simulink model "LoadFlow58BusNetwork_2023"  (R2023b)
settings: Solver=FixedStepDiscrete  StartTime=0.0  StopTime=4.5  FixedStep=75e-6  RelTol=1e-3  EnableMultiTasking=on
undefined symbols (not defined in the file): D1, D11, Delta
libraries: spsSeriesRLCBranchLib x41, spsLoadFlowBusLib x29, spsDistributedParametersLineLib x19, spsThreePhaseSeriesRLCLoadLib x15, spsThreePhaseTransformerTwoWindingsLib x13, spsThreePhaseParallelRLCLoadLib x11, spsThreePhaseVIMeasurementLib x11, spsSynchronousMachinepuStandardLib x7, spsExcitationSystemLib x7, spsHydraulicTurbineandGovernorLib x7, spsGenericPowerSystemStabilizerLib x7, spsMultiBandPowerSystemStabilizerLib x7
(part 3 of 5)

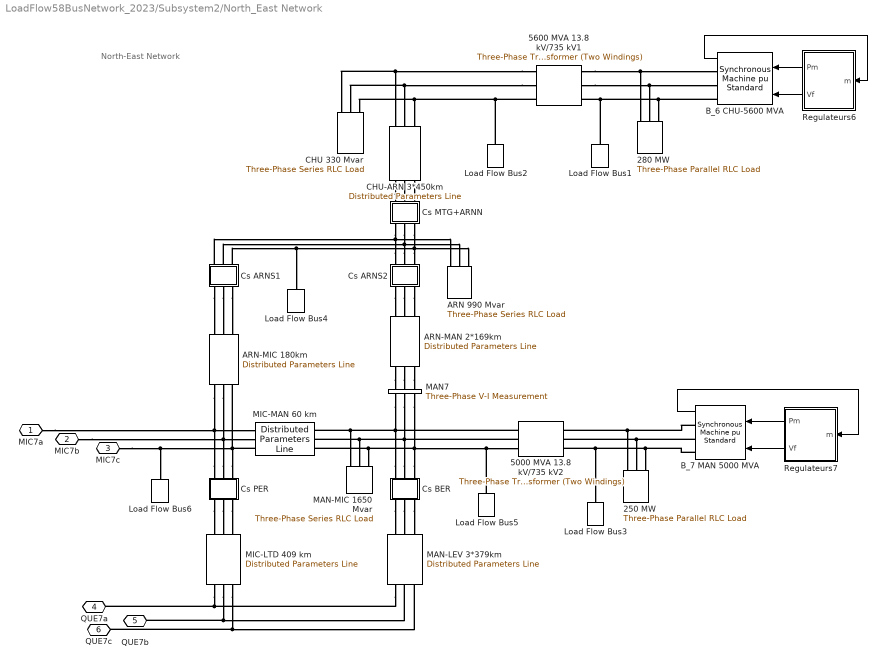
== system LoadFlow58BusNetwork_2023/Subsystem2/North_East Network ==
  note: North-East Network
  250 MW : spsThreePhaseParallelRLCLoadLib/Three-Phase Parallel RLC Load  LConnTagsString=A|B|C  Configuration=Y (grounded)  NominalVoltage=(13800)*1  Vabc=[1e3 1e3 1e3]  Vabcp=[1e3 1e3 1e3]  NominalFrequency=60  UnbalancedPower=off  ActivePower=250000000  InductivePower=0  CapacitivePower=0  Pabc=[10e3 9e3 11e3]  QLabc=[100 90 110]  QCabc=[100 90 110]  Pabcp=[10e3 9e3 11e3]  QLabcp=[100 90 110]  QCabcp=[100 90 110]  Measurements=None  LoadType=constant PQ
  280 MW : spsThreePhaseParallelRLCLoadLib/Three-Phase Parallel RLC Load  LConnTagsString=A|B|C  Configuration=Y (grounded)  NominalVoltage=(13800)*1  Vabc=[1e3 1e3 1e3]  Vabcp=[1e3 1e3 1e3]  NominalFrequency=60  UnbalancedPower=off  ActivePower=280000000  InductivePower=0  CapacitivePower=0  Pabc=[10e3 9e3 11e3]  QLabc=[100 90 110]  QCabc=[100 90 110]  Pabcp=[10e3 9e3 11e3]  QLabcp=[100 90 110]  QCabcp=[100 90 110]  Measurements=None  LoadType=constant PQ
  5000 MVA 13.8 kV/735 kV2 : spsThreePhaseTransformerTwoWindingsLib/Three-Phase Transformer (Two Windings)  Winding1Connection=Delta (D1)  Winding2Connection=Yg  CoreType=Three single-phase transformers  SetSaturation=off  Hysteresis=off  DataFile='basic_model'  SetInitialFlux=off  Measurements=None  UNITS=pu  NominalPower=[ 5000e6 60 ]  Winding1="[ 13.8e3 0.002  0.0]"  Winding2=[ 735e3 0.002 0.12]  Rm=500  Lm=500  L0=0.5  Saturation="[ 0,0  ;  0.005,1.2  ;  1.0,1.4 ]"  InitialFluxes=[ 0.8 , -0.8 , 0.7 ]  BreakLoop=off  DiscreteSolver=Trapezoidal iterative  DataType=off  TransfoNumber=0
  5600 MVA 13.8 kV/735 kV1 : spsThreePhaseTransformerTwoWindingsLib/Three-Phase Transformer (Two Windings)  Winding1Connection=Delta (D1)  Winding2Connection=Yg  CoreType=Three single-phase transformers  SetSaturation=off  Hysteresis=off  DataFile='basic_model'  SetInitialFlux=off  Measurements=None  UNITS=pu  NominalPower=[ 5600e6 60 ]  Winding1="[ 13.8e3 0.002  0.0]"  Winding2=[ 735e3 0.002 0.12]  Rm=500  Lm=500  L0=0.5  Saturation="[ 0,0  ;  0.005,1.2  ;  1.0,1.4 ]"  InitialFluxes=[ 0.8 , -0.8 , 0.7 ]  BreakLoop=off  DiscreteSolver=Trapezoidal iterative  DataType=off  TransfoNumber=0
  ARN 990 Mvar : spsThreePhaseSeriesRLCLoadLib/Three-Phase Series RLC Load  LConnTagsString=A|B|C  Configuration=Y (grounded)  NominalVoltage=735e3  Vabc=[1e3 1e3 1e3]  Vabcp=[1e3 1e3 1e3]  NominalFrequency=60  UnbalancedPower=off  ActivePower=3300000  InductivePower=990e6  CapacitivePower=0  Pabc=[10e3 9e3 11e3]  QLabc=[100 90 110]  QCabc=[100 90 110]  Pabcp=[10e3 9e3 11e3]  QLabcp=[100 90 110]  QCabcp=[100 90 110]  Measurements=None  LoadType=constant Z
  ARN-MAN 2*169km : spsDistributedParametersLineLib/Distributed Parameters Line  Phases=3  Length=169  Frequency=60  Resistance="[0.01273  0.3864]/2"  Inductance="[0.9337e-3  4.1264e-3]/2"  Capacitance=[12.74e-9 7.751e-9]*2  x1=[-0.000975 1.67050882449748e-09 347873.977312553 -681165.145140791;-0.0009 1.59985900326383e-09 366991.883229444 -671058.367402093;-0.000825 1.52793027922164e-09 385816.421450045 -660415.155872031;-0.00075 1.45478015109235e-09 404332.543926528 -649244.018571055;-0.000675 1.38046709396916e-09 422525.449153892 -637553.8855354;-0.0006 1.30505051257291e-09 440380.594002059 -625354.10167855;-0.000525 1.22859069376485e-09 457883.705341429 -612654.419321056;-0.00045 1.15114875835426e-09 475020.791452605 -599464.990394684;-0.000375 1.07278661223941e-09 491778.153211155 -585796.358327113;-0.0003 9.93566896920918e-10 508142.395038487 -571659.44961368;-0.000225 9.13552939427113e-10 524100.435610064 -557065.565082908;-0.00015 8.3280870169136e-10 539639.51831242 -542026.370862799;-7.5e-05 7.51398729421874e-10 554747.221440599 -526553.889055102]  x2=[-0.000975 1.50504449601884e-09 232985.418240298 -689450.364518884;-0.0009 1.46263645773588e-09 252383.458947633 -682588.200672076;-0.000825 1.41905921024769e-09 271579.748179482 -675180.3862616;-0.00075 1.37434758853916e-09 290558.940715946 -667232.842980953;-0.000675 1.32853733439658e-09 309305.864880903 -658751.923974632;-0.0006 1.28166506783619e-09 327805.534670012 -649744.408759529;-0.000525 1.2337682578307e-09 346043.161730299 -640217.497805485;-0.00045 1.18488519235719e-09 364004.167181736 -630178.806779352;-0.000375 1.13505494779026e-09 381674.193271379 -619636.360457139;-0.0003 1.08431735766499e-09 399039.114850732 -608598.586309131;-0.000225 1.03271298083461e-09 416085.050667176 -597074.307763098;-0.00015 9.80283069048393e-10 432798.374460432 -585072.737150982;-7.5e-05 9.27069533975612e-10 449165.725855181 -572603.4683447]  x3=[-0.000975 -5.34124314733807e-12 1583.75858462539 -1421.24992657659;-0.0009 -5.43018616572326e-12 1623.30400424483 -1375.9090252372;-0.000825 -5.5147883763722e-12 1661.55177948066 -1329.46824327516;-0.00075 -5.59498214957216e-12 1698.47133564656 -1281.96470474099;-0.000675 -5.67070337964786e-12 1734.03315981423 -1233.43638323657;-0.0006 -5.74189153620653e-12 1768.20882440555 -1183.9220715596;-0.000525 -5.80848971252505e-12 1800.97100991713 -1133.46135069323;-0.00045 -5.87044467104025e-12 1832.29352675917 -1082.09455816567;-0.000375 -5.92770688590623e-12 1862.15133619095 -1029.86275580491;-0.0003 -5.98023058258458e-12 1890.52057033645 -976.807696914584;-0.000225 -6.0279737744358e-12 1917.37855126396 -922.971792897006;-0.00015 -6.07089829628284e-12 1942.70380911446 -868.398079350128;-7.5e-05 -6.10896983491968e-12 1966.47609926432 -813.130181665554]  x4=[-0.000975 9.21214000394156e-12 1569.30174481224 -9115.59279820432;-0.0009 9.04527834437803e-12 1826.37892659041 -9067.5841614058;-0.000825 8.87118602770341e-12 2081.9961289992 -9012.32703656734;-0.00075 8.69000222065193e-12 2335.94901555807 -8949.86559538908;-0.000675 8.50187175878676e-12 2588.03458021512 -8880.2497685914;-0.0006 8.30694503072062e-12 2838.05130962701 -8803.53520600108;-0.000525 8.10537785789743e-12 3085.79934424562 -8719.78323206569;-0.00045 7.89733137003109e-12 3331.08063808276 -8629.06079683175;-0.000375 7.68297187630076e-12 3573.69911702505 -8531.44042242588;-0.0003 7.46247073240593e-12 3813.46083557263 -8427.00014508173;-0.000225 7.23600420358725e-12 4050.17413187616 -8315.82345275904;-0.00015 7.0037533237228e-12 4283.6497809484 -8197.99921840457;-7.5e-05 6.76590375061238e-12 4513.7011459278 -8073.62162890851]  x5=0.000955765248222805  V1=ones(3,3)  V2=ones(3,3)  I1=ones(3,3)  I2=ones(3,3)  nHarmo=1  Measurements=None  Decoupling=on  VsMag0=[624500.54274601 624501.904306242 624500.0432619]  VrMag0=[594207.380493356 594208.101305703 594207.286862308]  VsAngle0=[18.1135948354225 -101.886530201485 138.113424134242]  VrAngle0=[9.73160889879617 -110.268441654027 129.731523430545]  IsMag0=[1744.35611857334 1744.39210598387 1744.37536737728]  IrMag0=[7582.44376493461 7582.4337899273 7582.40838117022]  IsAngle0=[39.1559168024789 -80.8440356055226 159.154916919434]  IrAngle0=[0.828149284036499 -119.172115933984 120.828081951982]
      settings: AttributesFormatString=\n  LibrarySourceBlock=sps_lib/Power Grid Elements/Distributed Parameters Line
  ARN-MIC 180km : spsDistributedParametersLineLib/Distributed Parameters Line  Phases=3  Length=180  Frequency=60  Resistance="[0.01273  0.3864]"  Inductance="[0.9337e-3  4.1264e-3]"  Capacitance=[12.74e-9 7.751e-9]  x1=[-0.00105 1.27410114359668e-09 336203.730988153 -674396.62729794;-0.000975 1.20660459291676e-09 355134.952563368 -664622.476598216;-0.0009 1.13814350098693e-09 373782.284691251 -654317.036859764;-0.000825 1.0687725945566e-09 392130.820979812 -643488.546093432;-0.00075 9.98547327666939e-10 410165.893889885 -632145.660429059;-0.000675 9.27523837321831e-10 427873.086460132 -620297.447195891;-0.0006 8.5575889861276e-10 445238.243831739 -607953.377674304;-0.000525 7.83309879333687e-10 462247.484563601 -595123.319524603;-0.00045 7.10234694122118e-10 478887.211728927 -581817.528898967;-0.000375 6.36591758163024e-10 495144.123784416 -568046.642242835;-0.0003 5.62439940492634e-10 511005.225203312 -553821.667792299;-0.000225 4.87838516939434e-10 526457.836863822 -539153.976774286;-0.00015 4.12847122739972e-10 541489.606184618 -524055.294316571;-7.5e-05 3.37525704867365e-10 556088.516999299 -508537.690074895]  x2=[-0.00105 4.36302610467453e-09 192165.57848685 -719334.039084997;-0.000975 4.3093865404647e-09 212424.764832704 -713613.931123378;-0.0009 4.25230211859025e-09 232514.142071759 -707323.371103878;-0.000825 4.1918184714646e-09 252417.651063227 -700467.387603928;-0.00075 4.12798394878983e-09 272119.381246555 -693051.461191837;-0.000675 4.06084957890668e-09 291603.583360081 -685081.520045713;-0.0006 3.99046902800322e-09 310854.682030753 -676563.935214563;-0.000525 3.91689855721501e-09 329857.288224845 -667505.515525378;-0.00045 3.84019697765071e-09 348596.211549717 -657913.502140259;-0.000375 3.76042560337947e-09 367056.472396776 -647795.562767943;-0.0003 3.67764820241733e-09 385223.313915954 -637159.785534355;-0.000225 3.59193094575207e-09 403082.213812102 -626014.672517082;-0.00015 3.50334235444717e-09 420618.895953893 -614369.132948945;-7.5e-05 3.41195324486706e-09 437819.341785944 -602232.476096092]  x3=[-0.00105 3.66209367040117e-12 149.00166074947 -364.54093553914;-0.000975 3.89569353874418e-12 159.247423691884 -360.183291873256;-0.0009 4.12617924927843e-12 169.365886680365 -355.537723194838;-0.000825 4.35336655525346e-12 179.348961170419 -350.607943100407;-0.00075 4.57707384661297e-12 189.188666845044 -345.397892380743;-0.000675 4.79712229517107e-12 198.877137994077 -339.911735870675;-0.0006 5.01333599756484e-12 208.406629801921 -334.153859119776;-0.000525 5.22554211586878e-12 217.769524538628 -328.128864886622;-0.00045 5.43357101575876e-12 226.958337649405 -321.841569459417;-0.000375 5.63725640211517e-12 235.965723737644 -315.296998805928;-0.0003 5.83643545195665e-12 244.784482436724 -308.5003845558;-0.000225 6.03094894459828e-12 253.407564165872 -301.457159818471;-0.00015 6.22064138893022e-12 261.828075765492 -294.172954840033;-7.5e-05 6.40536114771486e-12 270.039286007448 -286.653592502493]  x4=[-0.00105 4.34965354391857e-12 1187.65933351948 -4979.46515427095;-0.000975 3.97419055552239e-12 1327.95758028668 -4943.89904376724;-0.0009 3.59555066000328e-12 1467.19427808263 -4904.38085601213;-0.000825 3.21403653630033e-12 1605.25812322151 -4860.94218124028;-0.00075 2.82995316096667e-12 1742.03874957796 -4813.61774366365;-0.000675 2.44360756437587e-12 1877.42681681208 -4762.44537371355;-0.0006 2.05530858528656e-12 2011.31409777444 -4707.46597779957;-0.000525 1.66536662396144e-12 2143.59356502117 -4648.72350560958;-0.00045 1.27409339403809e-12 2274.15947637011 -4586.26491497706;-0.000375 8.81801673349837e-13 2402.90745942944 -4520.14013434371;-0.0003 4.88805053895921e-13 2529.73459503142 -4450.40202284743;-0.000225 9.54176911608898e-14 2654.53949950437 -4377.10632806753;-0.00015 -2.98045947016516e-13 2777.22240571723 -4300.31164146093;-7.5e-05 -6.91271331824133e-13 2897.6852428319 -4220.07935152513]  x5=0.00101797482059234  V1=ones(3,3)  V2=ones(3,3)  I1=ones(3,3)  I2=ones(3,3)  nHarmo=1  Measurements=None  Decoupling=on  VsMag0=[615273.936100182 615275.237959051 615273.425867036]  VrMag0=[607930.231675994 607930.97680853 607930.152146888]  VsAngle0=[19.1774103741915 -100.822714483789 139.177242954875]  VrAngle0=[7.63692875074741 -112.363120449619 127.636843332413]  IsMag0=[322.896150601901 322.910343515413 322.909058922171]  IrMag0=[4197.50413399043 4197.49907033619 4197.48826872784]  IsAngle0=[14.9112658694072 -105.087543385455 134.90968031067]  IrAngle0=[6.09512812442914 -113.905082032173 126.095082904965]
      settings: AttributesFormatString=\n  LibrarySourceBlock=sps_lib/Power Grid Elements/Distributed Parameters Line
  "B_6 CHU-5600 MVA " : spsSynchronousMachinepuStandardLib/Synchronous Machine pu Standard  PresetModel=No  MechanicalLoad=Mechanical power Pm  ShowDetailedParameters=on  RotorType=Salient-pole  Units=per unit standard parameters  MeasurementBus=off  NominalParameters="[ 5600E6  13800   60 ]"  Reactances1=[ 31 32 33 34 35 36 37 ]  Reactances2=[ 1.305, 0.296, 0.252, 0.474, 0.243, 0.18 ]  dAxisTimeConstants=Short-circuit  qAxisTimeConstants=Open-circuit  TimeConstants1=[]  TimeConstants2=[]  TimeConstants3=[]  TimeConstants4=[]  TimeConstants5=[ 1.01, 0.053, 0.1 ]  TimeConstants6=[]  TimeConstants7=[]  TimeConstants8=[]  StatorResistance=2.8544e-3  Mechanical="[ 4.0 0  32]"  PolePairs=32  InitialConditions=[0 -61.7964 0.894782 0.894782 0.894782 8.48442 -111.516 128.484 1.31361]  SetSaturation=off  Saturation=[0.6404,0.7127,0.8441,0.9214,0.9956,1.082,1.19,1.316,1.457;0.7,0.7698,0.8872,0.9466,0.9969,1.046,1.1,1.151,1.201]  LoadFlowParameters=[1 5000000000 0 0 0]  TsPowergui=0  TsBlock=-1  IterativeModel=Trapezoidal non iterative  IterativeDiscreteModel=Trapezoidal non iterative  BusType=PV  Pref=5000000000  Qref=0  Qmin=-Inf  Qmax=Inf  PLF=0  QLF=0
  B_7 MAN 5000 MVA : spsSynchronousMachinepuStandardLib/Synchronous Machine pu Standard  PresetModel=No  MechanicalLoad=Mechanical power Pm  ShowDetailedParameters=on  RotorType=Salient-pole  Units=per unit standard parameters  MeasurementBus=off  NominalParameters="[ 5000E6  13800   60 ]"  Reactances1=[ 31 32 33 34 35 36 37 ]  Reactances2=[ 1.305, 0.296, 0.252, 0.474, 0.243, 0.18 ]  dAxisTimeConstants=Short-circuit  qAxisTimeConstants=Open-circuit  TimeConstants1=[]  TimeConstants2=[]  TimeConstants3=[]  TimeConstants4=[]  TimeConstants5=[ 1.01, 0.053, 0.1 ]  TimeConstants6=[]  TimeConstants7=[]  TimeConstants8=[]  StatorResistance=2.8544e-3  Mechanical="[ 3.7 0  32]"  PolePairs=32  InitialConditions=[0 -81.9543 0.907703 0.907703 0.907703 -8.76021 -128.76 111.24 1.25655]  SetSaturation=off  Saturation=[0.6404,0.7127,0.8441,0.9214,0.9956,1.082,1.19,1.316,1.457;0.7,0.7698,0.8872,0.9466,0.9969,1.046,1.1,1.151,1.201]  LoadFlowParameters=[1 4500000000 0 0 0]  TsPowergui=0  TsBlock=-1  IterativeModel=Trapezoidal non iterative  IterativeDiscreteModel=Trapezoidal non iterative  BusType=PV  Pref=4500000000  Qref=0  Qmin=-Inf  Qmax=Inf  PLF=0  QLF=0
  CHU 330 Mvar : spsThreePhaseSeriesRLCLoadLib/Three-Phase Series RLC Load  LConnTagsString=A|B|C  Configuration=Y (grounded)  NominalVoltage=735e3  Vabc=[1e3 1e3 1e3]  Vabcp=[1e3 1e3 1e3]  NominalFrequency=60  UnbalancedPower=off  ActivePower=1100000  InductivePower=330e6  CapacitivePower=0  Pabc=[10e3 9e3 11e3]  QLabc=[100 90 110]  QCabc=[100 90 110]  Pabcp=[10e3 9e3 11e3]  QLabcp=[100 90 110]  QCabcp=[100 90 110]  Measurements=None  LoadType=constant Z
  CHU-ARN 3*450km : spsDistributedParametersLineLib/Distributed Parameters Line  Phases=3  Length=450  Frequency=60  Resistance="[0.01273  0.3864]/3"  Inductance="[0.9337e-3  4.1264e-3]/3"  Capacitance=[12.74e-9 7.751e-9]*3  x1=[-0.00255 1.72762635052858e-09 0 0;-0.002475 1.64166254069958e-09 0 0;-0.0024 1.55438641095382e-09 0 0;-0.002325 1.46586772849405e-09 0 0;-0.00225 1.37617725380066e-09 0 0;-0.002175 1.28538668406679e-09 0 0;-0.0021 1.19356859588476e-09 0 0;-0.002025 1.10079638722939e-09 0 0;-0.00195 1.00714421878482e-09 0 0;-0.001875 9.1268695466157e-10 0 0;-0.0018 8.17500102551347e-10 0 0;-0.001725 7.21659753367315e-10 0 0;-0.00165 6.25242520418204e-10 0 0;-0.001575 5.28325478164804e-10 336692.129653582 -649852.524072734;-0.0015 4.30986100607809e-10 354929.318552025 -640074.408280408;-0.001425 3.33302199356297e-10 372882.782383818 -629784.626799569;-0.00135 2.35351861426314e-10 390538.169424672 -618991.405124095;-0.001275 1.37213386819311e-10 407881.366228322 -607703.37119025;-0.0012 3.89652259303204e-11 424898.508908603 -595929.548479649;-0.001125 -5.93140831640912e-11 441575.994222027 -583679.348806022;-0.00105 -1.57545977487958e-10 457900.49044201 -570962.564791552;-0.000975 -2.55651931967954e-10 473858.948016046 -557789.362038808;-0.0009 -3.53553522205142e-10 489438.609997323 -544170.271004514;-0.000825 -4.51172487166228e-10 504627.02224243 -530116.178581664;-0.00075 -5.48430791744245e-10 519412.043367009 -515638.319396704;-0.000675 -6.45250689138613e-10 533781.854451391 -500748.26682875;-0.0006 -7.41554783004751e-10 547724.968488461 -485457.923757998;-0.000525 -8.37266089323524e-10 561230.239566194 -469779.513050749;-0.00045 -9.32308097941092e-10 574286.871777528 -453725.567788636;-0.000375 -1.02660483372996e-09 586884.427850448 -437308.921249866;-0.0003 -1.12008091732232e-09 599012.837491376 -420542.696650499;-0.000225 -1.21266162536719e-09 610662.405435218 -403440.29665395;-0.00015 -1.30427295026308e-09 621823.819195603 -386015.392657098;-7.5e-05 -1.39484165931859e-09 632488.156509146 -368281.91386159]  x2=[-0.00255 2.63808008356907e-09 0 0;-0.002475 2.61305583763278e-09 0 0;-0.0024 2.58594275484099e-09 0 0;-0.002325 2.55676250897723e-09 0 0;-0.00225 2.52553842628357e-09 0 0;-0.002175 2.49229546681398e-09 0 0;-0.0021 2.45706020448161e-09 0 0;-0.002025 2.41986080581606e-09 0 0;-0.00195 2.38072700744746e-09 0 0;-0.001875 2.33969009233544e-09 0 0;-0.0018 2.29678286476207e-09 0 0;-0.001725 2.25203962410857e-09 0 0;-0.00165 2.20549613743692e-09 0 0;-0.001575 2.15718961089822e-09 24661.2186380232 -733238.396736893;-0.0015 2.10715865999068e-09 45380.4401578436 -732248.159297754;-0.001425 2.05544327869095e-09 66063.3852481457 -730672.573883845;-0.00135 2.00208480748357e-09 86693.5202790842 -728512.899994039;-0.001275 1.94712590031401e-09 107254.353836367 -725770.864038599;-0.0012 1.89061049049177e-09 127729.44990424 -722448.657959113;-0.001125 1.83258375557074e-09 148102.441004185 -718548.93747629;-0.00105 1.77309208123497e-09 168357.041278835 -714074.819967015;-0.000975 1.71218302421869e-09 188477.059510635 -709029.88197237;-0.0009 1.64990527429013e-09 208446.412064859 -703418.156338598;-0.000825 1.58630861532969e-09 228249.135746615 -697244.128993306;-0.00075 1.5214438855335e-09 247869.400561584 -690512.735359491;-0.000675 1.45536293677408e-09 267291.522370273 -683229.356410228;-0.0006 1.3881185931508e-09 286499.975425677 -675399.814367211;-0.000525 1.31976460876309e-09 305479.404784322 -667030.368046552;-0.00045 1.25035562474021e-09 324214.638580774 -658127.707855584;-0.000375 1.17994712556199e-09 342690.700155795 -648698.950444647;-0.0003 1.1085953947054e-09 360892.820028455 -638751.633018152;-0.000225 1.03635746965235e-09 378806.447702629 -628293.70730945;-0.00015 9.63291096294867e-10 396417.263298444 -617333.533224341;-7.5e-05 8.89454682773854e-10 413711.188999364 -605879.872158292]  x3=[-0.00255 3.59038620383718e-12 0 0;-0.002475 3.52504738676694e-12 0 0;-0.0024 3.45689070075075e-12 0 0;-0.002325 3.38597062920058e-12 0 0;-0.00225 3.31234386453652e-12 0 0;-0.002175 3.23606926286771e-12 0 0;-0.0021 3.15720779694368e-12 0 0;-0.002025 3.07582250741368e-12 0 0;-0.00195 2.99197845243291e-12 0 0;-0.001875 2.90574265565607e-12 0 0;-0.0018 2.81718405265965e-12 0 0;-0.001725 2.7263734358359e-12 0 0;-0.00165 2.63338339780246e-12 0 0;-0.001575 2.53828827337292e-12 -336.540930617731 -2064.60581280802;-0.0015 2.44116408013477e-12 -278.039507494979 -2073.29664773844;-0.001425 2.34208845768202e-12 -219.315823844082 -2080.33012105116;-0.00135 2.24114060555135e-12 -160.416822479249 -2085.70061029524;-0.001275 2.13840121991121e-12 -101.389586360986 -2089.40382238373;-0.0012 2.03395242905451e-12 -42.2813009586987 -2091.43679702556;-0.001125 1.92787772774653e-12 16.8607834686495 -2091.7979090919;-0.00105 1.82026191048052e-12 75.9893896436714 -2090.4868699153;-0.000975 1.7111910036942e-12 135.057251063289 -2087.50472752041;-0.0009 1.60075219700164e-12 194.017149782852 -2082.85386578623;-0.000825 1.48903377349512e-12 252.82195416144 -2076.53800254048;-0.00075 1.37612503917304e-12 311.424656538177 -2068.56218658759;-0.000675 1.26211625155008e-12 369.778410809435 -2058.9327936728;-0.0006 1.14709854750665e-12 427.836569876891 -2047.65752138548;-0.000525 1.03116387043554e-12 485.552722936506 -2034.74538300578;-0.00045 9.14404896743738e-13 542.880732578612 -2020.20670029955;-0.000375 7.96914961768345e-13 599.774771669448 -2004.0530952673;-0.0003 6.78787985165722e-13 656.189359984673 -1986.29748085374;-0.000225 5.60118395833562e-13 712.079400565561 -1966.95405062535;-0.00015 4.41001056425872e-13 767.400215768816 -1946.03826742429;-7.5e-05 3.21531187521218e-13 822.107582981203 -1923.56685100764]  x4=[-0.00255 2.00437993745201e-11 0 0;-0.002475 1.98906770635163e-11 0 0;-0.0024 1.97216544496055e-11 0 0;-0.002325 1.95368666468791e-11 0 0;-0.00225 1.93364613718792e-11 0 0;-0.002175 1.91205988255165e-11 0 0;-0.0021 1.88894515650076e-11 0 0;-0.002025 1.8643204365936e-11 0 0;-0.00195 1.83820540745448e-11 0 0;-0.001875 1.81062094503813e-11 0 0;-0.0018 1.78158909994174e-11 0 0;-0.001725 1.75113307977809e-11 0 0;-0.00165 1.7192772306237e-11 0 0;-0.001575 1.68604701755697e-11 -291.743024303822 -14207.2379327607;-0.0015 1.65146900430179e-11 110.022151992755 -14209.8063832451;-0.001425 1.6155708319929e-11 511.699378264424 -14201.015731924;-0.00135 1.57838119707997e-11 912.967559882371 -14180.8730059096;-0.001275 1.53992982838814e-11 1313.50592920182 -14149.3943069889;-0.0012 1.50024746335321e-11 1712.99430197878 -14106.6047987523;-0.001125 1.45936582345063e-11 2111.11333332043 -14052.5386864778;-0.00105 1.41731758883784e-11 2507.54477296454 -13987.2391897883;-0.000975 1.37413637223021e-11 2901.97171968386 -13910.7585081025;-0.0009 1.32985669203161e-11 3294.07887461213 -13823.1577789071;-0.000825 1.2845139447409e-11 3683.55279328913 -13724.5070288846;-0.00075 1.23814437665647e-11 4070.08213622342 -13614.8851179352;-0.000675 1.1907850549016e-11 4453.35791777235 -13494.3796761373;-0.0006 1.14247383779346e-11 4833.07375314048 -13363.0870336972;-0.000525 1.09324934457982e-11 5208.92610329886 -13221.1121439444;-0.00045 1.0431509245674e-11 5580.61451762951 -13068.5684994336;-0.000375 9.92218625666625e-12 5947.84187410102 -12905.5780412202;-0.0003 9.40493162377947e-12 6310.31461678342 -12732.2710613825;-0.000225 8.88015883245292e-12 6667.7429905122 -12548.7860988687;-0.00015 8.3482873780267e-12 7019.84127251426 -12355.2698287503;-7.5e-05 7.80974243040356e-12 7366.32800081025 -12151.8769449727]  x5=0.00254493705148084  V1=ones(3,3)  V2=ones(3,3)  I1=ones(3,3)  I2=ones(3,3)  nHarmo=1  Measurements=None  Decoupling=on  VsMag0=[597589.636778481 597591.191030954 597588.179734064]  VrMag0=[599025.218159133 599025.681050634 599025.146419324]  VsAngle0=[31.4089201475988 -88.5913271983184 151.408667420075]  VrAngle0=[5.94632207994051 -114.053711405452 125.946266994121]  IsMag0=[1726.12548309326 1726.16866029049 1726.16794416619]  IrMag0=[11726.0675753691 11726.049206287 11726.016456175]  IsAngle0=[-5.2389877445288 -125.238187761841 114.760171100696]  IrAngle0=[2.84375678806587 -117.156479810908 122.843716218949]
      settings: AttributesFormatString=\n  LibrarySourceBlock=sps_lib/Power Grid Elements/Distributed Parameters Line
  "Cs ARNS1 " : Subsystem  mask{Xc=25}
      mask prompts: Xc "Condensator Reactance at  60Hz  (ohm):"
      mask help: Series Compensation
      mask init:
      | Cs=1/Xc/(2*pi*60);
      mask Display: disp('Cs')
  Cs ARNS2 : Subsystem  mask{Xc=25/2}
      mask prompts: Xc "Condensator Reactance at  60Hz  (ohm):"
      mask help: Series Compensation
      mask init:
      | Cs=1/Xc/(2*pi*60);
      mask Display: disp('Cs')
  Cs BER : Subsystem  mask{Xc=22/3}
      mask prompts: Xc "Condensator Reactance at  60Hz  (ohm):"
      mask help: Series Compensation
      mask init:
      | Cs=1/Xc/(2*pi*60);
      mask Display: disp('Cs')
  "Cs MTG+ARNN " : Subsystem  mask{Xc=(30+25)/3}
      mask prompts: Xc "Condensator Reactance at  60Hz  (ohm):"
      mask help: Series Compensation
      mask init:
      | Cs=1/Xc/(2*pi*60);
      mask Display: disp('Cs')
  "Cs PER " : Subsystem  mask{Xc=22}
      mask prompts: Xc "Condensator Reactance at  60Hz  (ohm):"
      mask help: Series Compensation
      mask init:
      | Cs=1/Xc/(2*pi*60);
      mask Display: disp('Cs')
  Load Flow Bus1 : spsLoadFlowBusLib/Load Flow Bus  LConnTagsString=a  Phases=single  Connectors=on one side  ID=CHU_13.8  Vbase=13.8e3  Vref=1  Vangle=0  VLF=1  VLFb=1  VLFc=1  angleLF=4.726  angleLFb=0  angleLFc=0
      settings: AttributesFormatString=%<ID>\n%<Vbase>V\n%<VLF>pu\n%<angleLF>deg.
  Load Flow Bus2 : spsLoadFlowBusLib/Load Flow Bus  LConnTagsString=a  Phases=single  Connectors=on one side  ID=CHU7  Vbase=735e3  Vref=1  Vangle=0  VLF=1.009  VLFb=1  VLFc=1  angleLF=28.97  angleLFb=0  angleLFc=0
      settings: AttributesFormatString=%<ID>\n%<Vbase>V\n%<VLF>pu\n%<angleLF>deg.
  Load Flow Bus3 : spsLoadFlowBusLib/Load Flow Bus  LConnTagsString=a  Phases=single  Connectors=on one side  ID=MAN_13.8  Vbase=13.8e3  Vref=1  Vangle=0  VLF=1  VLFb=1  VLFc=1  angleLF=-16.23  angleLFb=0  angleLFc=0
      settings: AttributesFormatString=%<ID>\n%<Vbase>V\n%<VLF>pu\n%<angleLF>deg.
  Load Flow Bus4 : spsLoadFlowBusLib/Load Flow Bus  LConnTagsString=a  Phases=single  Connectors=on one side  ID=ARN7  Vbase=735e3  Vref=1  Vangle=0  VLF=1.054  VLFb=1  VLFc=1  angleLF=12.72  angleLFb=0  angleLFc=0
      settings: AttributesFormatString=%<ID>\n%<Vbase>V\n%<VLF>pu\n%<angleLF>deg.
  Load Flow Bus5 : spsLoadFlowBusLib/Load Flow Bus  LConnTagsString=a  Phases=single  Connectors=on one side  ID=MAN7  Vbase=735e3  Vref=1  Vangle=0  VLF=1.016  VLFb=1  VLFc=1  angleLF=7.996  angleLFb=0  angleLFc=0
      settings: AttributesFormatString=%<ID>\n%<Vbase>V\n%<VLF>pu\n%<angleLF>deg.
  Load Flow Bus6 : spsLoadFlowBusLib/Load Flow Bus  LConnTagsString=a  Phases=single  Connectors=on one side  ID=MIC7  Vbase=735e3  Vref=1  Vangle=0  VLF=1.041  VLFb=1  VLFc=1  angleLF=5.981  angleLFb=0  angleLFc=0
      settings: AttributesFormatString=%<ID>\n%<Vbase>V\n%<VLF>pu\n%<angleLF>deg.
  MAN-LEV 3*379km : spsDistributedParametersLineLib/Distributed Parameters Line  Phases=3  Length=379  Frequency=60  Resistance="[0.01273  0.3864]/3"  Inductance="[0.9337e-3  4.1264e-3]/3"  Capacitance=[12.74e-9 7.751e-9]*3  x1=[-0.002175 3.13627888012798e-09 -30838.3336725814 -721772.96842406;-0.0021 3.09617634025594e-09 -10421.0500052741 -722356.328523315;-0.002025 3.05359876439058e-09 10004.5640899602 -722362.24802597;-0.00195 3.0085801883946e-09 30422.1806897359 -721790.722200066;-0.001875 2.96115659942884e-09 50815.4782637432 -720642.207914604;-0.0018 2.91136590718471e-09 71168.1547219292 -718917.623274331;-0.001725 2.85924791357977e-09 91463.94044614 -716618.34688582;-0.00165 2.80484428094067e-09 111686.611295803 -713746.216755438;-0.001575 2.74819849869895e-09 131820.001577259 -710303.528820064;-0.0015 2.68935584862621e-09 151848.016966368 -706293.03511176;-0.001425 2.62836336863661e-09 171754.647374066 -701717.941557834;-0.00135 2.56526981518542e-09 191523.979744588 -696581.905418071;-0.001275 2.50012562429392e-09 211140.210776117 -690889.032361177;-0.0012 2.43298287123157e-09 230587.659553705 -684643.873182771;-0.001125 2.36389522888783e-09 249850.780084356 -677851.420167544;-0.00105 2.29291792486694e-09 268914.173724252 -670517.10309851;-0.000975 2.22010769733973e-09 287762.601488198 -662646.784916515;-0.0009 2.14552274968805e-09 306380.996231429 -654246.757033494;-0.000825 2.06922270397787e-09 324754.47469406 -645323.73430321;-0.00075 1.99126855329829e-09 342868.34939853 -635884.84965351;-0.000675 1.91172261300465e-09 360708.140390553 -625937.64838436;-0.0006 1.8306484709045e-09 378259.586814167 -615490.08213626;-0.000525 1.74811093642657e-09 395508.658311648 -604550.502533813;-0.00045 1.66417598881306e-09 412441.566239159 -593127.654509574;-0.000375 1.57891072437684e-09 429044.774689187 -581230.669313478;-0.0003 1.49238330286569e-09 445305.011310934 -568869.05721346;-0.000225 1.40466289297646e-09 461209.277920033 -556052.699893093;-0.00015 1.31581961706265e-09 476744.860889102 -542791.842552324;-7.5e-05 1.22592449507968e-09 491899.341310817 -529097.085717612]  x2=[-0.002175 1.35614139967261e-08 -379192.175232082 -624794.196144324;-0.0021 1.36303727731618e-08 -361377.320734359 -635264.451513561;-0.002025 1.36884356381543e-08 -343273.586735698 -645226.886200131;-0.00195 1.37355561771378e-08 -324895.445084063 -654673.536386174;-0.001875 1.37716967226743e-08 -306257.586984696 -663596.850564071;-0.0018 1.37968283845648e-08 -287374.91125619 -671989.695573;-0.001725 1.38109310729432e-08 -268262.51242061 -679845.362301074;-0.00165 1.38139935143362e-08 -248935.668637155 -687157.571048508;-0.001575 1.3806013260675e-08 -229409.829489035 -693920.47654751;-0.0015 1.37869966912524e-08 -209700.60363331 -700128.672634898;-0.001425 1.37569590076229e-08 -189823.746323567 -705777.19657371;-0.00135 1.37159242214512e-08 -169795.146815414 -710861.533020334;-0.001275 1.36639251353176e-08 -149630.815664849 -715377.617634008;-0.0012 1.36010033164958e-08 -129346.87192967 -719321.84032579;-0.001125 1.35272090637252e-08 -108959.530284144 -722691.048144409;-0.00105 1.34426013670023e-08 -88485.0880572454 -725482.547796685;-0.000975 1.33472478604253e-08 -67939.9122048211 -727694.107800508;-0.0009 1.32412247681284e-08 -47340.4262260959 -729323.960268648;-0.000825 1.31246168433494e-08 -26703.0970349784 -730370.80232198;-0.00075 1.29975173006792e-08 -6044.42179666215 -730833.797130983;-0.000675 1.28600277415475e-08 14619.0852599556 -730712.574584693;-0.0006 1.27122580730043e-08 35270.906043496 -730007.231586556;-0.000525 1.25543264198615e-08 55894.5318044082 -728718.331976975;-0.00045 1.23863590302664e-08 76473.476331811 -726846.906082576;-0.000375 1.22084901747801e-08 96991.2891323175 -724394.449892584;-0.0003 1.20208620390443e-08 117431.568580308 -721362.923862956;-0.000225 1.18236246101198e-08 137777.975029139 -717754.751349214;-0.00015 1.16169355565895e-08 158014.243872805 -713572.81666926;-7.5e-05 1.14009601025203e-08 178124.198547619 -708820.46279769]  x3=[-0.002175 3.74838767807378e-12 -359.273937220667 349.81481958126;-0.0021 5.31546885815293e-12 -369.020063583087 339.517457527932;-0.002025 6.87830093375627e-12 -378.471200952874 328.948690413848;-0.00195 8.43563460083471e-12 -387.619794235424 318.11696674973;-0.001875 9.98622495068278e-12 -396.458530185244 307.030945249746;-0.0018 1.15288324650996e-11 -404.980343252052 295.69948790986;-0.001725 1.30622240072409e-11 -413.178421228872 284.131652923692;-0.00165 1.45851738073696e-11 -421.046210697604 272.336687441538;-0.001575 1.60964644427173e-11 -428.577422267726 260.324020178334;-0.0015 1.75948878106736e-11 -435.766035603943 248.10325387649;-0.001425 1.90792460945249e-11 -442.606304238741 235.684157629604;-0.00135 2.05483527209705e-11 -449.092760166035 223.076659073198;-0.001275 2.20010333086513e-11 -455.220218212201 210.290836448717;-0.0012 2.34361266069322e-11 -460.983780181032 197.336910547135;-0.001125 2.48524854241883e-11 -466.378838769274 184.225236538619;-0.00105 2.62489775448521e-11 -471.40108124964 170.966295694754;-0.000975 2.76244866344894e-11 -476.046492918333 157.570687009982;-0.0009 2.89779131321799e-11 -480.311360304343 144.049118728928;-0.000825 3.03081751294894e-11 -484.192274137935 130.412399786386;-0.00075 3.16142092353311e-11 -487.686132075972 116.671431166833;-0.000675 3.28949714260237e-11 -490.790141181876 102.837197190337;-0.0006 3.41494378798682e-11 -493.50182015826 88.9207567318689;-0.000525 3.53766057955756e-11 -495.81900133044 74.9332343810027;-0.00045 3.65754941938901e-11 -497.739832379242 60.8858115490893;-0.000375 3.77451447017699e-11 -499.262777821714 46.7897175310078;-0.0003 3.88846223184951e-11 -500.386620238573 32.6562205286386;-0.000225 3.99930161630936e-11 -501.110461247385 18.4966186432357;-0.00015 4.10694402024851e-11 -501.433722220723 4.32223084389724;-7.5e-05 4.21130339597621e-11 -501.356144748711 -9.85561208064552]  x4=[-0.002175 5.06161336107903e-11 -7842.63207577848 -13937.1348474401;-0.0021 4.98967373509418e-11 -7445.48599612148 -14153.2795346848;-0.002025 4.91374544027007e-11 -7042.38810887894 -14358.110306822;-0.00195 4.83388917252383e-11 -6633.66064433432 -14551.4634252663;-0.001875 4.75016876773406e-11 -6219.63033296903 -14733.1843264933;-0.0018 4.66265115071138e-11 -5800.62814427909 -14903.127745595;-0.001725 4.57140628169978e-11 -5376.98902220321 -15061.1578324024;-0.00165 4.47650710045145e-11 -4949.05161737366 -15207.148260082;-0.001575 4.37802946791988e-11 -4517.15801640422 -15340.9823261196;-0.0015 4.27605210561774e-11 -4081.6534684313 -15462.5530456107;-0.001425 4.17065653268817e-11 -3642.88610912711 -15571.7632367821;-0.00135 4.06192700073955e-11 -3201.2066824053 -15668.525598678;-0.001275 3.94995042649611e-11 -2756.96826004169 -15752.7627809467;-0.0012 3.83481632231799e-11 -2310.52595943403 -15824.4074456738;-0.001125 3.71661672464647e-11 -1862.23665972663 -15883.4023212103;-0.00105 3.59544612043141e-11 -1412.45871652662 -15929.7002479555;-0.000975 3.47140137159985e-11 -961.551675439962 -15963.264216055;-0.0009 3.34458163762605e-11 -509.875984656192 -15984.0673949863;-0.000825 3.21508829626496e-11 -57.7927068116533 -15992.0931550065;-0.00075 3.08302486251232e-11 394.336769638453 -15987.3350804459;-0.000675 2.94849690585646e-11 846.151019308466 -15969.7969748363;-0.0006 2.81161196588757e-11 1297.28886880019 -15939.4928578712;-0.000525 2.67247946633226e-11 1747.38968541938 -15896.4469541979;-0.00045 2.53121062758186e-11 2196.09366546 -15840.6936740532;-0.000375 2.3879183777846e-11 2643.04212182582 -15772.2775857562;-0.0003 2.24271726257252e-11 3087.87777075934 -15691.2533800811;-0.000225 2.09572335349545e-11 3530.24501744904 -15597.6858265382;-0.00015 1.94705415523525e-11 3969.79024028635 -15491.6497215981;-7.5e-05 1.79682851167428e-11 4406.1620735454 -15373.2298289008]  x5=0.00214340253891386  V1=ones(3,3)  V2=ones(3,3)  I1=ones(3,3)  I2=ones(3,3)  nHarmo=1  Measurements=None  Decoupling=on  VsMag0=[589863.022608742 589863.802580103 589862.857709067]  VrMag0=[596743.737336247 596743.91108333 596743.706580376]  VsAngle0=[14.5334919446077 -105.466570291732 134.533395214781]  VrAngle0=[-14.273856882172 -134.273869923449 105.726122150014]  IsMag0=[413.109398330103 413.092934230975 413.107596304933]  IrMag0=[13174.4675205298 13174.4678533391 13174.4493337434]  IsAngle0=[-117.256344753987 122.744684998152 2.74614766448615]  IrAngle0=[-12.3870102586412 -132.387102424571 107.612942404917]
      settings: AttributesFormatString=\n  LibrarySourceBlock=sps_lib/Power Grid Elements/Distributed Parameters Line
  MAN-MIC 1650 Mvar : spsThreePhaseSeriesRLCLoadLib/Three-Phase Series RLC Load  LConnTagsString=A|B|C  Configuration=Y (grounded)  NominalVoltage=735e3  Vabc=[1e3 1e3 1e3]  Vabcp=[1e3 1e3 1e3]  NominalFrequency=60  UnbalancedPower=off  ActivePower=5500000  InductivePower=1650e6  CapacitivePower=0  Pabc=[10e3 9e3 11e3]  QLabc=[100 90 110]  QCabc=[100 90 110]  Pabcp=[10e3 9e3 11e3]  QLabcp=[100 90 110]  QCabcp=[100 90 110]  Measurements=None  LoadType=constant Z
  MAN7 : spsThreePhaseVIMeasurementLib/Three-Phase V-I Measurement  VoltageMeasurement=no  SetLabelV=on  LabelV=Vabc_MAN7  Vpu=on  VpuLL=off  CurrentMeasurement=no  SetLabelI=on  LabelI=Iabc_MAN7  Ipu=on  Pbase=100e6  Vbase=735e3  OutputType=Magnitude  PhasorSimulation=off  PSBequivalent=0
  MIC-LTD 409 km : spsDistributedParametersLineLib/Distributed Parameters Line  Phases=3  Length=409  Frequency=60  Resistance="[0.01273  0.3864]"  Inductance="[0.9337e-3  4.1264e-3]"  Capacitance=[12.74e-9 7.751e-9]  x1=[-0.002325 4.49009478615413e-09 0 0;-0.00225 4.49931280977409e-09 0 0;-0.002175 4.5049341515757e-09 0 0;-0.0021 4.50695431794436e-09 0 0;-0.002025 4.50537169398996e-09 0 0;-0.00195 4.50018754483788e-09 0 0;-0.001875 4.49140601461764e-09 0 0;-0.0018 4.47903412315013e-09 0 0;-0.001725 4.46308176033609e-09 0 0;-0.00165 4.44356167825028e-09 0 0;-0.001575 4.42048948094765e-09 0 0;-0.0015 4.39388361198971e-09 0 0;-0.001425 4.36376533970102e-09 138503.934059133 -724390.238526699;-0.00135 4.33015874016762e-09 158927.516108489 -720185.156863837;-0.001275 4.29309067799098e-09 179224.05393314 -715404.370205781;-0.0012 4.25259078481284e-09 199377.322791297 -710051.700240236;-0.001125 4.20869143562815e-09 219371.212468191 -704131.425809675;-0.00105 4.16142772290495e-09 239189.740154329 -697648.279490894;-0.000975 4.11083742853204e-09 258817.063221914 -690607.443811864;-0.0009 4.05696099361669e-09 278237.491889193 -683014.547108899;-0.000825 3.99984148615662e-09 297435.501762632 -674875.659027448;-0.00075 3.93952456661215e-09 316395.746246877 -666197.285670115;-0.000675 3.87605845140587e-09 335103.068812591 -656986.364395777;-0.0006 3.80949387437923e-09 353542.515112344 -647250.25827397;-0.000525 3.73988404623661e-09 371699.344934899 -636996.750198959;-0.00045 3.66728461200958e-09 389559.043988303 -626234.036668217;-0.000375 3.59175360657504e-09 407107.335502396 -614970.721230264;-0.0003 3.51335140826308e-09 424330.19164144 -603215.807607127;-0.000225 3.43214069059144e-09 441213.844717755 -590978.6924969;-0.00015 3.34818637216525e-09 457744.798197401 -578269.158062169;-7.5e-05 3.26155556478212e-09 473909.837489099 -565097.364110297]  x2=[-0.002325 1.33910378738474e-08 0 0;-0.00225 1.3481614433438e-08 0 0;-0.002175 1.35614139967261e-08 0 0;-0.0021 1.36303727731618e-08 0 0;-0.002025 1.36884356381543e-08 0 0;-0.00195 1.37355561771378e-08 0 0;-0.001875 1.37716967226743e-08 0 0;-0.0018 1.37968283845648e-08 0 0;-0.001725 1.38109310729432e-08 0 0;-0.00165 1.38139935143362e-08 0 0;-0.001575 1.3806013260675e-08 0 0;-0.0015 1.37869966912524e-08 0 0;-0.001425 1.37569590076229e-08 -189823.746323567 -705777.19657371;-0.00135 1.37159242214512e-08 -169795.146815414 -710861.533020335;-0.001275 1.36639251353176e-08 -149630.815664849 -715377.617634008;-0.0012 1.36010033164958e-08 -129346.87192967 -719321.84032579;-0.001125 1.35272090637252e-08 -108959.530284144 -722691.048144409;-0.00105 1.34426013670023e-08 -88485.0880572454 -725482.547796685;-0.000975 1.33472478604253e-08 -67939.9122048211 -727694.107800508;-0.0009 1.32412247681284e-08 -47340.4262260959 -729323.960268648;-0.000825 1.31246168433494e-08 -26703.0970349784 -730370.80232198;-0.00075 1.29975173006792e-08 -6044.42179666215 -730833.797130983;-0.000675 1.28600277415475e-08 14619.0852599556 -730712.574584693;-0.0006 1.27122580730043e-08 35270.906043496 -730007.231586556;-0.000525 1.25543264198615e-08 55894.5318044082 -728718.331976975;-0.00045 1.23863590302664e-08 76473.476331811 -726846.906082576;-0.000375 1.22084901747801e-08 96991.2891323175 -724394.449892584;-0.0003 1.20208620390443e-08 117431.568580308 -721362.923862956;-0.000225 1.18236246101198e-08 137777.975029139 -717754.751349214;-0.00015 1.16169355565895e-08 158014.243872805 -713572.81666926;-7.5e-05 1.14009601025203e-08 178124.198547619 -708820.46279769]  x3=[-0.002325 2.872105047819e-12 0 0;-0.00225 3.36341134358248e-12 0 0;-0.002175 3.85202897977983e-12 0 0;-0.0021 4.33756736294876e-12 0 0;-0.002025 4.81963836113476e-12 0 0;-0.00195 5.2978566141578e-12 0 0;-0.001875 5.77183984166341e-12 0 0;-0.0018 6.24120914871171e-12 0 0;-0.001725 6.70558932866023e-12 0 0;-0.00165 7.16460916309837e-12 0 0;-0.001575 7.61790171859373e-12 0 0;-0.0015 8.06510464001305e-12 0 0;-0.001425 8.50586044018339e-12 -163.959464483914 -404.071950170223;-0.00135 8.93981678566187e-12 -152.470711052349 -408.545860687912;-0.001275 9.36662677838567e-12 -140.860074867249 -412.693185895529;-0.0012 9.78594923297703e-12 -129.136837293531 -416.510610484759;-0.001125 1.01974489494816e-11 -117.310369707941 -419.995082864793;-0.00105 1.06007969813221e-11 -105.390126007715 -423.143817601725;-0.000975 1.09956708982535e-11 -93.3856350532816 -425.954297645184;-0.0009 1.13817550441081e-11 -81.3064930510346 -428.424276340424;-0.000825 1.17587407891272e-11 -69.1623558822736 -430.551779224269;-0.00075 1.21263267766742e-11 -56.96293138444 -432.335105603466;-0.000675 1.2484219164135e-11 -44.7179715908196 -433.772829914192;-0.0006 1.28321318578109e-11 -32.4372649349175 -434.863802861632;-0.000525 1.31697867416179e-11 -20.1306284257332 -435.607152338703;-0.00045 1.34969138994081e-11 -7.80789980019433 -436.002284123208;-0.000375 1.38132518307369e-11 4.52107034097995 -436.048882352843;-0.0003 1.4118547659902e-11 16.8464264076984 -435.746909777697;-0.000225 1.44125573380888e-11 29.1583156989054 -435.096607790026;-0.00015 1.46950458384591e-11 41.4468962786799 -434.098496231288;-7.5e-05 1.49657873440278e-11 53.7023448437281 -432.753372976594]  x4=[-0.002325 1.51256191642448e-11 0 0;-0.00225 1.50337331831171e-11 0 0;-0.002175 1.49298294657066e-11 0 0;-0.0021 1.48139910710553e-11 0 0;-0.002025 1.46863105986035e-11 0 0;-0.00195 1.45468901141673e-11 0 0;-0.001875 1.43958410683486e-11 0 0;-0.0018 1.42332842074437e-11 0 0;-0.001725 1.40593494769199e-11 0 0;-0.00165 1.38741759175395e-11 0 0;-0.001575 1.36779115542127e-11 0 0;-0.0015 1.34707132776684e-11 0 0;-0.001425 1.32527467190389e-11 -1447.81766818147 -4750.17763764053;-0.00135 1.30241861174559e-11 -1312.94851541747 -4789.2095920444;-0.001275 1.27852141807674e-11 -1177.02981169903 -4824.41312557774;-0.0012 1.25360219394831e-11 -1040.17020835828 -4855.7600970745;-0.001125 1.2276808594068e-11 -902.479108868109 -4883.22544824528;-0.00105 1.20077813557042e-11 -764.066581386699 -4906.78722370858;-0.000975 1.17291552806499e-11 -625.043270770739 -4926.42658854161;-0.0009 1.14411530983263e-11 -485.520310127607 -4942.12784333662;-0.000825 1.11440050332715e-11 -345.609231977269 -4953.87843675076;-0.00075 1.0837948621102e-11 -205.421879094888 -4961.66897553944;-0.000675 1.05232285186311e-11 -65.0703151054172 -4965.49323206515;-0.0006 1.02000963082931e-11 75.3332650983386 -4965.34814927575;-0.000525 9.86881029703295e-12 215.676625042613 -4961.23384314819;-0.00045 9.52963530981924e-12 355.847576392791 -4953.15360259584;-0.000375 9.18284247794717e-12 495.734068635051 -4941.11388683936;-0.0003 8.82870902230043e-12 635.22427864783 -4925.12432024333;-0.000225 8.46751803174503e-12 774.206700091515 -4905.19768462262;-0.00015 8.09955823683244e-12 912.570232544907 -4881.34990902486;-7.5e-05 7.72512377899271e-12 1050.2042703172 -4853.60005699699]  x5=0.00231306500901259  V1=ones(3,3)  V2=ones(3,3)  I1=ones(3,3)  I2=ones(3,3)  nHarmo=1  Measurements=None  Decoupling=on  VsMag0=[602176.302414453 602177.107483075 602176.16572093]  VrMag0=[596743.737336247 596743.91108333 596743.706580376]  VsAngle0=[11.6043495452569 -108.395709698231 131.604253585458]  VrAngle0=[-14.273856882172 -134.273869923449 105.726122150014]  IsMag0=[359.486265157156 359.489496854291 359.491918798638]  IrMag0=[4093.84062560462 4093.84102057872 4093.83505039147]  IsAngle0=[-21.3064747486809 -141.305731641554 98.6934507450032]  IrAngle0=[-16.1707432095108 -136.170836500555 103.829205357655]
      settings: AttributesFormatString=\n  LibrarySourceBlock=sps_lib/Power Grid Elements/Distributed Parameters Line
  MIC-MAN 60 km : spsDistributedParametersLineLib/Distributed Parameters Line  Phases=3  Length=60  Frequency=60  Resistance="[0.01273  0.3864]"  Inductance="[0.9337e-3  4.1264e-3]"  Capacitance=[12.74e-9 7.751e-9]  x1=[-0.000375 3.76042560337947e-09 367056.472396776 -647795.562767943;-0.0003 3.67764820241733e-09 385223.313915954 -637159.785534355;-0.000225 3.59193094575207e-09 403082.213812102 -626014.672517082;-0.00015 3.50334235444717e-09 420618.895953893 -614369.132948945;-7.5e-05 3.41195324486706e-09 437819.341785944 -602232.476096092]  x2=[-0.000375 1.13505494779026e-09 381674.193271379 -619636.360457139;-0.0003 1.08431735766499e-09 399039.114850732 -608598.586309131;-0.000225 1.03271298083461e-09 416085.050667176 -597074.307763098;-0.00015 9.80283069048393e-10 432798.374460432 -585072.737150982;-7.5e-05 9.27069533975612e-10 449165.725855181 -572603.4683447]  x3=[-0.000375 -1.24503734806182e-11 2615.73591803648 -3083.53120523849;-0.0003 -1.31153616437878e-11 2701.86358792152 -3008.35057124458;-0.000225 -1.3769865587531e-11 2785.83142939427 -2930.76510783332;-0.00015 -1.44133621114096e-11 2867.57231984701 -2850.83683563707;-7.5e-05 -1.50453368141482e-11 2947.0209168626 -2768.62964809369]  x4=[-0.000375 2.14630546878962e-11 -38.3285845652442 -1696.07516225689;-0.0003 2.19506180969483e-11 9.63578970455663 -1696.48092157512;-0.000225 2.24206345177495e-11 57.5924612715001 -1695.53054000167;-0.00015 2.28727282263645e-11 105.503094306097 -1693.22477725703;-7.5e-05 2.33065378259997e-11 153.329389781358 -1689.56547653267]  x5=0.000339324940197445  V1=ones(3,3)  V2=ones(3,3)  I1=ones(3,3)  I2=ones(3,3)  nHarmo=1  Measurements=None  Decoupling=on  VsMag0=[607930.231675994 607930.97680853 607930.152146888]  VrMag0=[594207.380493356 594208.101305703 594207.286862308]  VsAngle0=[7.63692875074741 -112.363120449619 127.636843332413]  VrAngle0=[9.73160889879617 -110.268441654027 129.731523430545]  IsMag0=[3306.19691878093 3306.20035207242 3306.19654855246]  IrMag0=[1387.14843174252 1387.15088256341 1387.14865267793]  IsAngle0=[18.4076953761291 -101.592346383782 138.407622969114]  IrAngle0=[-23.1945765462604 -143.194624454311 96.8053118315442]
      settings: AttributesFormatString=\n  LibrarySourceBlock=sps_lib/Power Grid Elements/Distributed Parameters Line
  Regulateurs6 : Subsystem
  Regulateurs7 : Subsystem
  "MIC7a " : PMIOPort  Side=Left
  MIC7b : PMIOPort  Port=2  Side=Left
  MIC7c : PMIOPort  Port=3  Side=Left
  QUE7a : PMIOPort  Port=4  Side=Left
  QUE7b : PMIOPort  Port=5  Side=Left
  QUE7c : PMIOPort  Port=6  Side=Left
  wires:
  Regulateurs6/1(Pm) -> "B_6 CHU-5600 MVA "/1
  Regulateurs6/2(Vf) -> "B_6 CHU-5600 MVA "/2
  "B_6 CHU-5600 MVA "/1 -> Regulateurs6/1(m)
  Regulateurs7/1(Pm) -> B_7 MAN 5000 MVA/1
  Regulateurs7/2(Vf) -> B_7 MAN 5000 MVA/2
  B_7 MAN 5000 MVA/1 -> Regulateurs7/1(m)
  connections:
  "Cs PER "/RConn3 -- MIC-LTD 409 km/LConn3
  "Cs PER "/RConn2 -- MIC-LTD 409 km/LConn2
  "Cs PER "/RConn1 -- MIC-LTD 409 km/LConn1
  Cs BER/RConn3 -- MAN-LEV 3*379km/LConn3
  Cs BER/RConn2 -- MAN-LEV 3*379km/LConn2
  Cs BER/RConn1 -- MAN-LEV 3*379km/LConn1
  Cs ARNS2/RConn3 -- ARN-MAN 2*169km/LConn3
  Cs ARNS2/RConn2 -- ARN-MAN 2*169km/LConn2
  Cs ARNS2/RConn1 -- ARN-MAN 2*169km/LConn1
  CHU-ARN 3*450km/RConn3 -- "Cs MTG+ARNN "/LConn3
  CHU-ARN 3*450km/RConn2 -- "Cs MTG+ARNN "/LConn2
  CHU-ARN 3*450km/RConn1 -- "Cs MTG+ARNN "/LConn1
  Load Flow Bus2/LConn1 -- 5600 MVA 13.8 kV/735 kV1/RConn3 -- CHU-ARN 3*450km/LConn3 -- CHU 330 Mvar/LConn3
  5600 MVA 13.8 kV/735 kV1/RConn2 -- CHU-ARN 3*450km/LConn2 -- CHU 330 Mvar/LConn2
  5600 MVA 13.8 kV/735 kV1/RConn1 -- CHU-ARN 3*450km/LConn1 -- CHU 330 Mvar/LConn1
  "B_6 CHU-5600 MVA "/RConn3 -- Load Flow Bus1/LConn1 -- 5600 MVA 13.8 kV/735 kV1/LConn3 -- 280 MW/LConn3
  5600 MVA 13.8 kV/735 kV1/LConn2 -- "B_6 CHU-5600 MVA "/RConn2 -- 280 MW/LConn2
  5600 MVA 13.8 kV/735 kV1/LConn1 -- "B_6 CHU-5600 MVA "/RConn1 -- 280 MW/LConn1
  "Cs ARNS1 "/RConn1 -- ARN-MIC 180km/LConn1
  "Cs ARNS1 "/RConn2 -- ARN-MIC 180km/LConn2
  "Cs ARNS1 "/RConn3 -- ARN-MIC 180km/LConn3
  "Cs PER "/LConn3 -- Load Flow Bus6/LConn1 -- MIC7c/RConn1 -- MIC-MAN 60 km/LConn3 -- ARN-MIC 180km/RConn3
  "Cs PER "/LConn2 -- MIC7b/RConn1 -- ARN-MIC 180km/RConn2 -- MIC-MAN 60 km/LConn2
  "Cs PER "/LConn1 -- "MIC7a "/RConn1 -- ARN-MIC 180km/RConn1 -- MIC-MAN 60 km/LConn1
  ARN-MAN 2*169km/RConn1 -- MAN7/LConn1
  ARN-MAN 2*169km/RConn2 -- MAN7/LConn2
  ARN-MAN 2*169km/RConn3 -- MAN7/LConn3
  Cs BER/LConn1 -- 5000 MVA 13.8 kV/735 kV2/RConn1 -- MIC-MAN 60 km/RConn1 -- MAN-MIC 1650 Mvar/LConn1 -- MAN7/RConn1
  Cs BER/LConn2 -- 5000 MVA 13.8 kV/735 kV2/RConn2 -- MIC-MAN 60 km/RConn2 -- MAN-MIC 1650 Mvar/LConn2 -- MAN7/RConn2
  Cs BER/LConn3 -- Load Flow Bus5/LConn1 -- 5000 MVA 13.8 kV/735 kV2/RConn3 -- MIC-MAN 60 km/RConn3 -- MAN-MIC 1650 Mvar/LConn3 -- MAN7/RConn3
  B_7 MAN 5000 MVA/RConn1 -- 5000 MVA 13.8 kV/735 kV2/LConn1 -- 250 MW/LConn1
  B_7 MAN 5000 MVA/RConn2 -- 5000 MVA 13.8 kV/735 kV2/LConn2 -- 250 MW/LConn2
  B_7 MAN 5000 MVA/RConn3 -- 5000 MVA 13.8 kV/735 kV2/LConn3 -- Load Flow Bus3/LConn1 -- 250 MW/LConn3
  MIC-LTD 409 km/RConn2 -- MAN-LEV 3*379km/RConn2 -- QUE7b/RConn1
  Cs ARNS2/LConn1 -- ARN 990 Mvar/LConn1 -- "Cs MTG+ARNN "/RConn1 -- "Cs ARNS1 "/LConn1
  Cs ARNS2/LConn2 -- ARN 990 Mvar/LConn2 -- "Cs MTG+ARNN "/RConn2 -- "Cs ARNS1 "/LConn2
  Cs ARNS2/LConn3 -- Load Flow Bus4/LConn1 -- "Cs ARNS1 "/LConn3 -- ARN 990 Mvar/LConn3 -- "Cs MTG+ARNN "/RConn3
  MIC-LTD 409 km/RConn1 -- QUE7a/RConn1 -- MAN-LEV 3*379km/RConn1
  MIC-LTD 409 km/RConn3 -- QUE7c/RConn1 -- MAN-LEV 3*379km/RConn3
